simulink model "SlidingMode_sign_prev"  (Simulink 8.5)
settings: Solver=ode23  StartTime=0.0  StopTime=10  RelTol=1e-3
undefined symbols (not defined in the file): magnitude
settings Model: Creator=tamzi  LastModifiedBy=Tamzid  CovExternalEMLEnable=on
settings SolverCC: ZeroCrossAlgorithm=Adaptive
settings OptimizationCC: ExpressionDepthLimit=128  InitFltsAndDblsToZero=on
settings DebuggingCC: SaveWithParameterizedLinksMsg=none  SignalResolutionControl=TryResolveAllWithWarning  IgnoredZcDiagnostic=none  SolverPrmCheckMsg=warning  MultiTaskDSMMsg=warning  MultiTaskCondExecSysMsg=none  FcnCallInpInsideContextMsg=EnableAllAsError  StateNameClashWarn=none
settings SFSimCC: SimUseLocalCustomCode=on
settings RTWCC: RTWUseLocalCustomCode=on
settings GRTTargetCC: TargetFcnLib=ansi_tfl_tmw.mat  GeneratePreprocessorConditionals=Use local settings

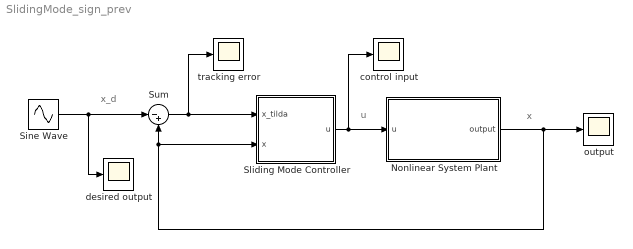
== system SlidingMode_sign_prev ==
  note: x_d
  note: x
  note: u
  Nonlinear System Plant : Subsystem
  Sine Wave : Sin  Frequency=pi/2  SampleTime=0
  Sliding Mode Controller : Subsystem
  Sum : Sum  Inputs=|-+
  control input : Scope
      settings: TimeRange=auto  MaxDataPoints=5000  SaveName=control_input  YMin=-12.9999  YMax=39.1288  SampleTime=-1  DataFormat=Array
  desired output : Scope
      settings: TimeRange=auto  LimitDataPoints=on  MaxDataPoints=5000  SaveName=desired_output  YMin=-1.24996  YMax=1.24984  SampleTime=-1  DataFormat=Array
  output : Scope
      settings: TimeRange=auto  MaxDataPoints=5000  SaveName=output  YMin=-1.30086  YMax=1.2982  SampleTime=-1  DataFormat=Array
  tracking error : Scope
      settings: TimeRange=auto  MaxDataPoints=5000  SaveName=tracking_error  YMin=-0.1544  YMax=0.09504  SampleTime=-1  DataFormat=Array
  wires:
  Sine Wave/1 -> desired output/1, Sum/1
  Sum/1 -> Sliding Mode Controller/1(x_tilda), tracking error/1
  Sliding Mode Controller/1(u) -> Nonlinear System Plant/1(u), control input/1
  Nonlinear System Plant/1(output) -> output/1, Sum/2, Sliding Mode Controller/2(x)

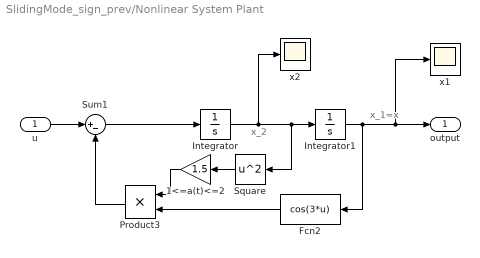
== system SlidingMode_sign_prev/Nonlinear System Plant ==
  note: x_1=x
  note: x_2
  u : Inport
  1<=a(t)<=2 : Gain  Gain=1.5
  Fcn2 : Fcn  Expr=cos(3*u)
  Integrator : Integrator
  Integrator1 : Integrator
  Product3 : Product  RndMeth=Zero
  Square : Math  Operator=square  SaturateOnIntegerOverflow=on
  Sum1 : Sum  Inputs=|+-
  x1 : Scope
      settings: TimeRange=auto  LimitDataPoints=on  MaxDataPoints=5000  SaveName=x1  YMin=-0.125568  YMax=-0.11361  SampleTime=-1  DataFormat=Array
  x2 : Scope
      settings: TimeRange=auto  LimitDataPoints=on  MaxDataPoints=5000  SaveName=x2  YMin=-0.125568  YMax=-0.11361  SampleTime=-1  DataFormat=Array
  output : Outport
  wires:
  Integrator/1 -> Square/1, Integrator1/1, x2/1
  Integrator1/1 -> Fcn2/1, output/1, x1/1
  Fcn2/1 -> Product3/2
  Product3/1 -> Sum1/2
  Sum1/1 -> Integrator/1
  u/1 -> Sum1/1
  Square/1 -> 1<=a(t)<=2/1
  1<=a(t)<=2/1 -> Product3/1

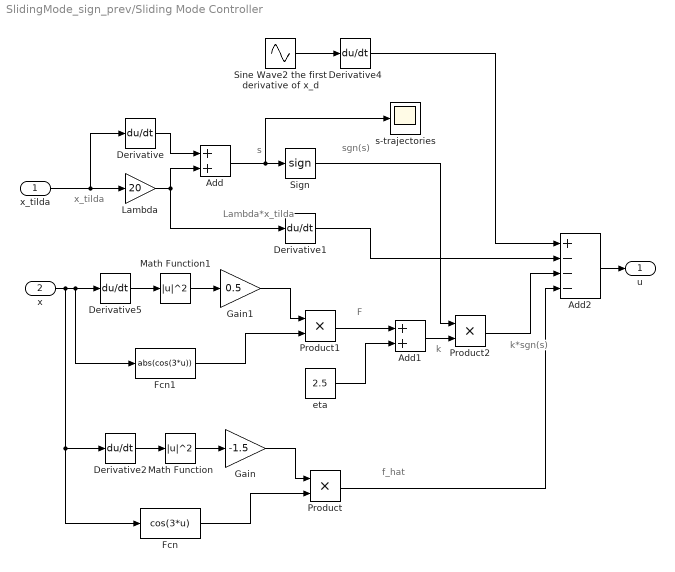
== system SlidingMode_sign_prev/Sliding Mode Controller ==
  note: x_tilda
  note: s
  note: sgn(s)
  note: Lambda*x_tilda
  note: F
  note: k
  note: f_hat
  note: k*sgn(s)
  x_tilda : Inport
  x : Inport  Port=2
  Add : Sum
  Add1 : Sum
  Add2 : Sum  Inputs=+---
  Derivative{,1..2,4..5} (5 alike) : Derivative
  Fcn : Fcn  Expr=cos(3*u)
  Fcn1 : Fcn  Expr=abs(cos(3*u))
  Gain : Gain  Gain=-1.5
  Gain1 : Gain  Gain=0.5
  Lambda : Gain  Gain=20
  Math Function : Math  Operator=magnitude^2  SaturateOnIntegerOverflow=on
  Math Function1 : Math  Operator=magnitude^2  SaturateOnIntegerOverflow=on
  Product : Product  RndMeth=Zero
  Product1 : Product  RndMeth=Zero
  Product2 : Product  RndMeth=Zero
  Sign : Signum
  Sine Wave2 the first derivative of x_d : Sin  Amplitude=-pi/2  Frequency=pi/2  Phase=pi/2  SampleTime=0
  eta : Constant  Value=2.5
  s-trajectories : Scope
      settings: TimeRange=auto  LimitDataPoints=on  MaxDataPoints=5000  SaveName=s_trajectories  YMin=-0.125568  YMax=-0.11361  SampleTime=-1  DataFormat=Array
  u : Outport
  wires:
  x_tilda/1 -> Lambda/1, Derivative/1
  Derivative/1 -> Add/1
  Lambda/1 -> Add/2, Derivative1/1
  Add/1 -> Sign/1, s-trajectories/1
  Sign/1 -> Product2/1
  Derivative1/1 -> Add2/2
  Sine Wave2 the first derivative of x_d/1 -> Derivative4/1
  Derivative4/1 -> Add2/1
  Derivative5/1 -> Math Function1/1
  Math Function1/1 -> Gain1/1
  Gain1/1 -> Product1/1
  Fcn1/1 -> Product1/2
  Product1/1 -> Add1/1
  eta/1 -> Add1/2
  Add1/1 -> Product2/2
  Derivative2/1 -> Math Function/1
  Math Function/1 -> Gain/1
  Gain/1 -> Product/1
  Fcn/1 -> Product/2
  Product/1 -> Add2/4
  Product2/1 -> Add2/3
  x/1 -> Fcn1/1, Derivative5/1, Derivative2/1, Fcn/1
  Add2/1 -> u/1
